simulink model "raspi_MODEL"  (R2022b)
settings: Solver=FixedStepAuto  StartTime=0.0  StopTime=1000  RelTol=1e-3  EnableMultiTasking=on
libraries: raspberrypiBasiclib x6, embedlinuxNetworklib x3, raspberrypiNetworklib x2, raspberrypiAVlib x1
settings Model: SimulationMode=external  Creator=Asus  LastModifiedBy=VIKAS CHEIIURU
settings SolverCC: PositivePriorityOrder=on
settings OptimizationCC: EnhancedBackFolding=on  PassReuseOutputArgsAs=Individual arguments  ZeroExternalMemoryAtStartup=off  ZeroInternalMemoryAtStartup=off  MaxStackSize=64  OptimizeBlockOrder=speed  DifferentSizesBufferReuse=on  OptimizationCustomize=off  EfficientTunableParamExpr=on
settings DebuggingCC: ParameterTunabilityLossMsg=error
settings HardwareCC: ProdBitPerPointer=32  ProdBitPerSizeT=32  ProdBitPerPtrDiffT=32  ProdLargestAtomicInteger=Long  ProdLargestAtomicFloat=Double  ProdWordSize=32  ProdLongLongMode=on  ProdHWDeviceType=ARM Compatible->ARM Cortex
settings RTWCC: Description=Embedded Coder  SystemTargetFile=ert.tlc  HardwareBoard=Raspberry Pi  TemplateMakefile=ert_default_tmf  Toolchain=GNU GCC Embedded Linux  BuildConfiguration=Faster Runs
settings CodeAppCC: ForceParamTrailComments=on  IgnoreCustomStorageClasses=off  OperatorAnnotations=on  SimulinkDataObjDesc=on  SFDataObjDesc=on  InsertBlockDesc=on
settings ERTTargetCC: SupportVariableSizeSignals=on  ExtMode=on  ExtModeTransport=2  ExtModeStaticAlloc=on  ExtModeMexFile=ext_xcp  ExtModeMexArgs='192.168.235.51' 0 17725  ExtModeIntrfLevel=Level2 - Open

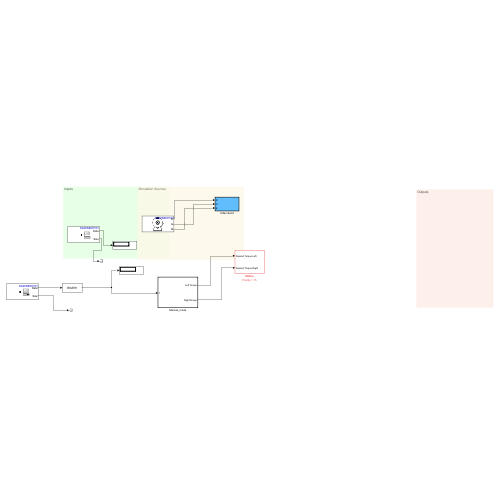
[thumbnail: Simulink's stored preview of the top-level diagram]
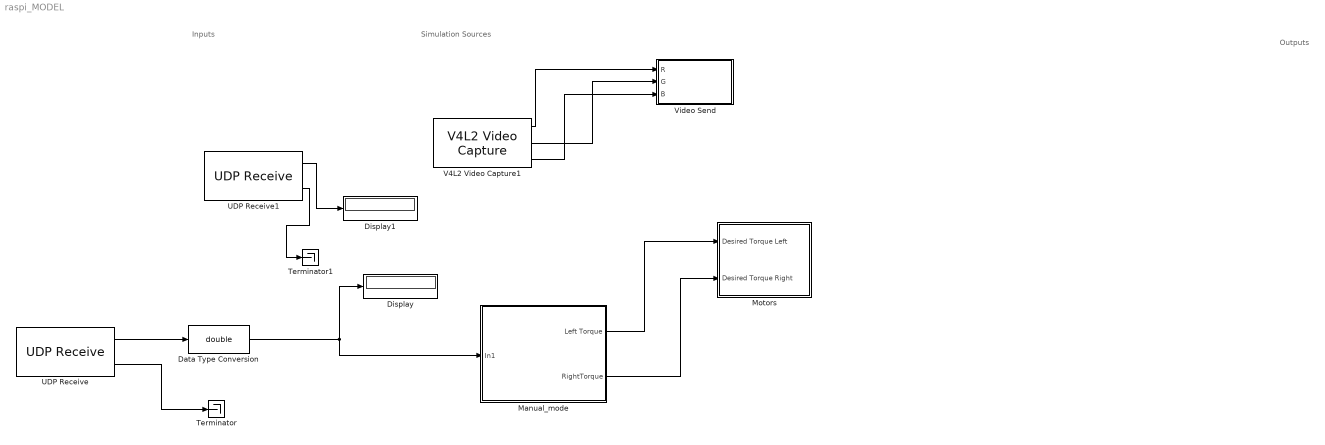
== system raspi_MODEL ==
  note: Inputs
  note: Outputs
  note: Simulation Sources
  Data Type Conversion : DataTypeConversion  OutDataTypeStr=double  RndMeth=Round  SaturateOnIntegerOverflow=off
  Display : Display
  Display1 : Display
  Manual_mode : Subsystem  TreatAsAtomicUnit=on
  Motors : Subsystem  Priority=15
      settings: AttributesFormatString=Priority = %<Priority>
  Terminator : Terminator
  Terminator1 : Terminator
  UDP Receive : raspberrypiNetworklib/UDP Receive  localURL='0.0.0.0'  localPort=26001  remoteURL='0.0.0.0'  remotePort=-1  recvBufferSize=8192  signalDatatype=double  dims=1  isVarSize=off  showBlockingTime=off  blockingTime=0  sampletime=0.01  blockPlatform=Raspberry Pi
  UDP Receive1 : raspberrypiNetworklib/UDP Receive  localURL='0.0.0.0'  localPort=26000  remoteURL='0.0.0.0'  remotePort=-1  recvBufferSize=8192  signalDatatype=boolean  dims=1  isVarSize=off  showBlockingTime=off  blockingTime=0  sampletime=0.01  blockPlatform=Raspberry Pi
  V4L2 Video Capture1 : raspberrypiAVlib/V4L2 Video Capture  DeviceName=/dev/video0  Resolution=160x120  CustomResolution=[ 320, 240 ]  PixelFormat=RGB  SampleTime=0.1  pixelOrder=planar  simOutput=Colorbars  imSizeSelection=320x240  imSize=[640, 480]  roi=[0, 0, 640, 480]  m_devName='/dev/video0'  blockPlatform=LINUX  HorizontalFlip=off  VerticalFlip=off  Brightness=0.5  Saturation=0.5  Contrast=0.5  Sharpness=0.5  CameraPan=0  CameraTilt=0  CameraZoom=0.5  EnableManualFocus=on  ManualFocus=0.5
  Video Send : Subsystem  TreatAsAtomicUnit=on
  wires:
  V4L2 Video Capture1/3 -> Video Send/3(B)
  V4L2 Video Capture1/2 -> Video Send/2(G)
  V4L2 Video Capture1/1 -> Video Send/1(R)
  Manual_mode/2(RightTorque) -> Motors/2(Desired Torque Right)
  Manual_mode/1(Left Torque) -> Motors/1(Desired Torque Left)
  UDP Receive1/1 -> Display1/1
  UDP Receive1/2 -> Terminator1/1
  UDP Receive/1 -> Data Type Conversion/1
  Data Type Conversion/1 -> Manual_mode/1(In1), Display/1
  UDP Receive/2 -> Terminator/1

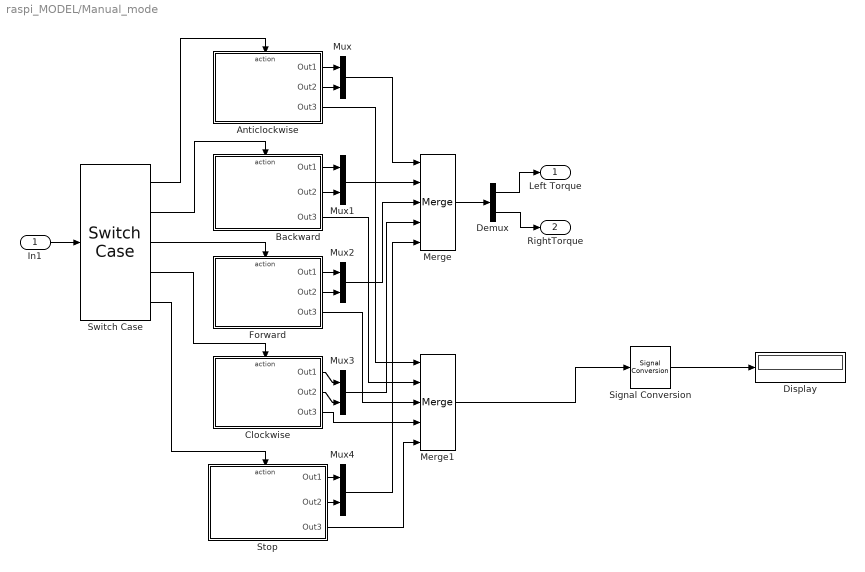
== system raspi_MODEL/Manual_mode ==
  In1 : Inport
  " Anticlockwise" : Subsystem  TreatAsAtomicUnit=on
  Backward : Subsystem  TreatAsAtomicUnit=on
  Clockwise : Subsystem  TreatAsAtomicUnit=on
  Demux : Demux  Outputs=2
  Display : Display
  Forward : Subsystem  TreatAsAtomicUnit=on
  Merge : Merge  Inputs=5
  Merge1 : Merge  Inputs=5  InitialOutput=5
  Mux{,1..4} (5 alike) : Mux  Inputs=2
  Signal Conversion : SignalConversion  OverrideOpt=off
  Stop : Subsystem  TreatAsAtomicUnit=on
  Switch Case : SwitchCase  Priority=1  CaseConditions={2, 3, 4, 5}
      settings: AttributesFormatString=Priority = %<Priority>
  Left Torque : Outport  VectorParamsAs1DForOutWhenUnconnected=off
  RightTorque : Outport  Port=2  VectorParamsAs1DForOutWhenUnconnected=off
  wires:
  Switch Case/1 -> " Anticlockwise"/Action
  Switch Case/2 -> Backward/Action
  Switch Case/3 -> Forward/Action
  Switch Case/4 -> Clockwise/Action
  Switch Case/5 -> Stop/Action
  " Anticlockwise"/2(Out2) -> Mux/2
  " Anticlockwise"/1(Out1) -> Mux/1
  Backward/2(Out2) -> Mux1/2
  Backward/1(Out1) -> Mux1/1
  Forward/2(Out2) -> Mux2/2
  Forward/1(Out1) -> Mux2/1
  Clockwise/1(Out1) -> Mux3/1
  Clockwise/2(Out2) -> Mux3/2
  Stop/1(Out1) -> Mux4/1
  Stop/2(Out2) -> Mux4/2
  Mux2/1 -> Merge/3
  Mux1/1 -> Merge/2
  Mux/1 -> Merge/1
  Mux3/1 -> Merge/4
  Mux4/1 -> Merge/5
  Merge/1 -> Demux/1
  Demux/1 -> Left Torque/1
  Demux/2 -> RightTorque/1
  Stop/3(Out3) -> Merge1/5
  Clockwise/3(Out3) -> Merge1/4
  Forward/3(Out3) -> Merge1/3
  Backward/3(Out3) -> Merge1/2
  " Anticlockwise"/3(Out3) -> Merge1/1
  In1/1 -> Switch Case/1
  Merge1/1 -> Signal Conversion/1
  Signal Conversion/1 -> Display/1

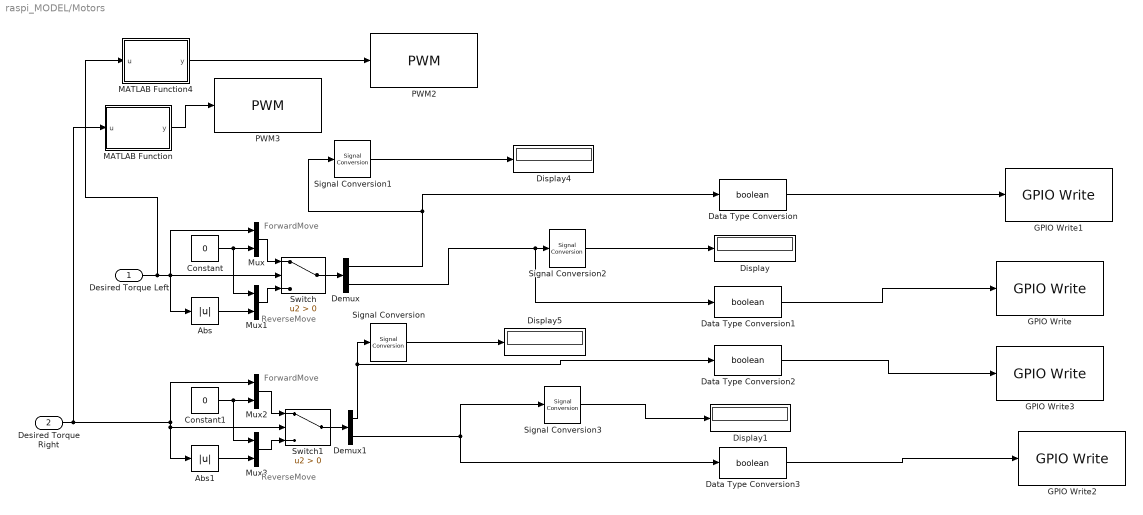
== system raspi_MODEL/Motors ==
  note: ReverseMove
  note: ForwardMove
  note: ReverseMove
  note: ForwardMove
  Desired Torque Left : Inport
  Desired Torque Right : Inport  Port=2
  Abs : Abs  OutDataTypeStr=int16  RndMeth=Round  SaturateOnIntegerOverflow=off
  Abs1 : Abs  OutDataTypeStr=int16  RndMeth=Round  SaturateOnIntegerOverflow=off
  Constant : Constant  Value=0  OutDataTypeStr=int16
  Constant1 : Constant  Value=0  OutDataTypeStr=int16
  Data Type Conversion : DataTypeConversion  OutDataTypeStr=boolean  RndMeth=Nearest  SaturateOnIntegerOverflow=off
  Data Type Conversion1 : DataTypeConversion  OutDataTypeStr=boolean  RndMeth=Round  SaturateOnIntegerOverflow=off
  Data Type Conversion2 : DataTypeConversion  OutDataTypeStr=boolean  RndMeth=Round  SaturateOnIntegerOverflow=off
  Data Type Conversion3 : DataTypeConversion  OutDataTypeStr=boolean  RndMeth=Round  SaturateOnIntegerOverflow=off
  Demux : Demux  Outputs=2
  Demux1 : Demux  Outputs=2
  Display{,1,4..5} (4 alike) : Display
  GPIO Write : raspberrypiBasiclib/GPIO Write  board=Pi 3 Model B  gpio=27  direction=Output  blockPlatform=Raspberry Pi
  GPIO Write1 : raspberrypiBasiclib/GPIO Write  board=Pi 3 Model B  gpio=22  direction=Output  blockPlatform=Raspberry Pi
  GPIO Write2 : raspberrypiBasiclib/GPIO Write  board=Pi 3 Model B  gpio=24  direction=Output  blockPlatform=Raspberry Pi
  GPIO Write3 : raspberrypiBasiclib/GPIO Write  board=Pi 3 Model B  gpio=23  direction=Output  blockPlatform=Raspberry Pi
  MATLAB Function : MATLAB Function  TreatAsAtomicUnit=on
  MATLAB Function4 : MATLAB Function  TreatAsAtomicUnit=on
  Mux{,1..3} (4 alike) : Mux  Inputs=2
  PWM2 : raspberrypiBasiclib/PWM  board=Pi 3 Model B  Pin_=12  Frequency=500  blockPlatform=Raspberry Pi
  PWM3 : raspberrypiBasiclib/PWM  board=Pi 3 Model B  Pin_=13  Frequency=500  blockPlatform=Raspberry Pi
  Signal Conversion{,1..3} (4 alike) : SignalConversion  OverrideOpt=off
  Switch : Switch  Criteria=u2 > Threshold  SaturateOnIntegerOverflow=off  InputSameDT=off
  Switch1 : Switch  Criteria=u2 > Threshold  SaturateOnIntegerOverflow=off  InputSameDT=off
  wires:
  Switch/1 -> Demux/1
  Mux1/1 -> Switch/3
  Constant/1 -> Mux/2, Mux1/1
  Mux/1 -> Switch/1
  Abs/1 -> Mux1/2
  Switch1/1 -> Demux1/1
  Mux3/1 -> Switch1/3
  Constant1/1 -> Mux2/2, Mux3/1
  Abs1/1 -> Mux3/2
  Mux2/1 -> Switch1/1
  Demux/1 -> Data Type Conversion/1, Signal Conversion1/1
  Demux/2 -> Data Type Conversion1/1, Signal Conversion2/1
  Demux1/2 -> Data Type Conversion3/1, Signal Conversion3/1
  Signal Conversion1/1 -> Display4/1
  Desired Torque Right/1 -> Abs1/1, Switch1/2, Mux2/1, MATLAB Function/1(u)
  Desired Torque Left/1 -> MATLAB Function4/1(u), Abs/1, Mux/1, Switch/2
  Signal Conversion/1 -> Display5/1
  Demux1/1 -> Data Type Conversion2/1, Signal Conversion/1
  Signal Conversion2/1 -> Display/1
  Signal Conversion3/1 -> Display1/1
  MATLAB Function/1(y) -> PWM3/1
  MATLAB Function4/1(y) -> PWM2/1
  Data Type Conversion/1 -> GPIO Write1/1
  Data Type Conversion1/1 -> GPIO Write/1
  Data Type Conversion2/1 -> GPIO Write3/1
  Data Type Conversion3/1 -> GPIO Write2/1

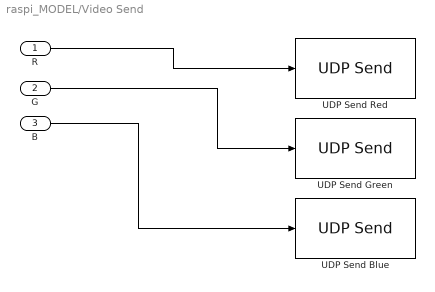
== system raspi_MODEL/Video Send ==
  R : Inport
  G : Inport  Port=2
  B : Inport  Port=3
  UDP Send Blue : embedlinuxNetworklib/UDP Send  remoteURL='255.255.255.255'  remotePort=25002  localURL='255.255.255.255'  localPortSource=Automatically determine  localPort=-1  sampletime=-1  blockPlatform=Raspberry Pi  separateLengthPort=0
  UDP Send Green : embedlinuxNetworklib/UDP Send  remoteURL='255.255.255.255'  remotePort=25001  localURL='255.255.255.255'  localPortSource=Automatically determine  localPort=-1  sampletime=-1  blockPlatform=Raspberry Pi  separateLengthPort=0
  UDP Send Red : embedlinuxNetworklib/UDP Send  remoteURL='255.255.255.255'  remotePort=2500  localURL='255.255.255.255'  localPortSource=Automatically determine  localPort=-1  sampletime=-1  blockPlatform=Raspberry Pi  separateLengthPort=0
  wires:
  R/1 -> UDP Send Red/1
  G/1 -> UDP Send Green/1
  B/1 -> UDP Send Blue/1

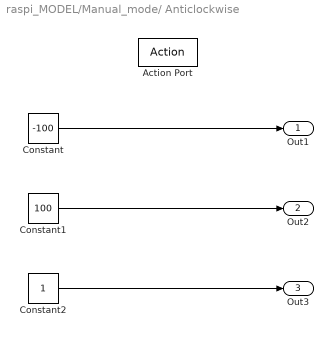
== system raspi_MODEL/Manual_mode/ Anticlockwise ==
  Action Port : ActionPort  ActionPortLabel=case [ 2 ]:
  Constant : Constant  Value=-100  OutDataTypeStr=int16
  Constant1 : Constant  Value=100  OutDataTypeStr=int16
  Constant2 : Constant  OutDataTypeStr=uint8
  Out1 : Outport  InitialOutput=80  VectorParamsAs1DForOutWhenUnconnected=off
  Out2 : Outport  Port=2  InitialOutput=120  VectorParamsAs1DForOutWhenUnconnected=off
  Out3 : Outport  Port=3  InitialOutput=120  VectorParamsAs1DForOutWhenUnconnected=off
  wires:
  Constant/1 -> Out1/1
  Constant1/1 -> Out2/1
  Constant2/1 -> Out3/1

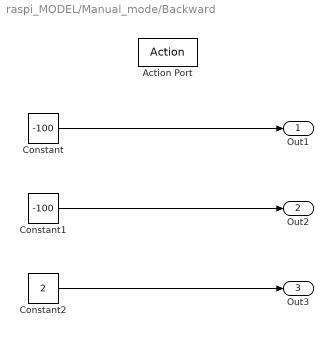
== system raspi_MODEL/Manual_mode/Backward ==
  Action Port : ActionPort  ActionPortLabel=case [ 3 ]:
  Constant : Constant  Value=-100  OutDataTypeStr=int16
  Constant1 : Constant  Value=-100  OutDataTypeStr=int16
  Constant2 : Constant  Value=2  OutDataTypeStr=uint8
  Out1 : Outport  InitialOutput=-100  VectorParamsAs1DForOutWhenUnconnected=off
  Out2 : Outport  Port=2  InitialOutput=-100  VectorParamsAs1DForOutWhenUnconnected=off
  Out3 : Outport  Port=3  InitialOutput=120  VectorParamsAs1DForOutWhenUnconnected=off
  wires:
  Constant/1 -> Out1/1
  Constant1/1 -> Out2/1
  Constant2/1 -> Out3/1

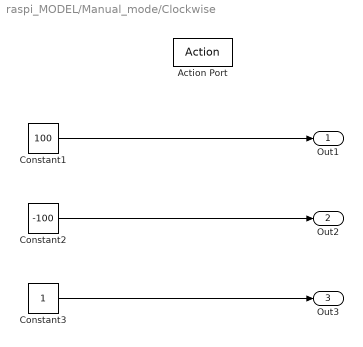
== system raspi_MODEL/Manual_mode/Clockwise ==
  Action Port : ActionPort  ActionPortLabel=case [ 5 ]:
  Constant1 : Constant  Value=100  OutDataTypeStr=int16
  Constant2 : Constant  Value=-100  OutDataTypeStr=int16
  Constant3 : Constant  OutDataTypeStr=uint8
  Out1 : Outport  InitialOutput=0  VectorParamsAs1DForOutWhenUnconnected=off
  Out2 : Outport  Port=2  InitialOutput=0  VectorParamsAs1DForOutWhenUnconnected=off
  Out3 : Outport  Port=3  InitialOutput=120  VectorParamsAs1DForOutWhenUnconnected=off
  wires:
  Constant1/1 -> Out1/1
  Constant2/1 -> Out2/1
  Constant3/1 -> Out3/1

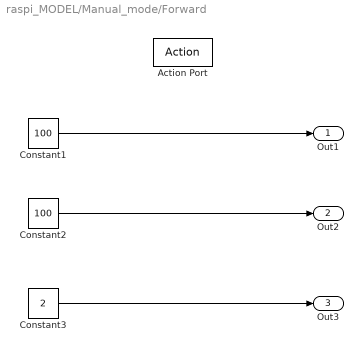
== system raspi_MODEL/Manual_mode/Forward ==
  Action Port : ActionPort  ActionPortLabel=case [ 4 ]:
  Constant1 : Constant  Value=100  OutDataTypeStr=int16
  Constant2 : Constant  Value=100  OutDataTypeStr=int16
  Constant3 : Constant  Value=2  OutDataTypeStr=uint8
  Out1 : Outport  InitialOutput=0  VectorParamsAs1DForOutWhenUnconnected=off
  Out2 : Outport  Port=2  InitialOutput=0  VectorParamsAs1DForOutWhenUnconnected=off
  Out3 : Outport  Port=3  InitialOutput=120  VectorParamsAs1DForOutWhenUnconnected=off
  wires:
  Constant1/1 -> Out1/1
  Constant2/1 -> Out2/1
  Constant3/1 -> Out3/1

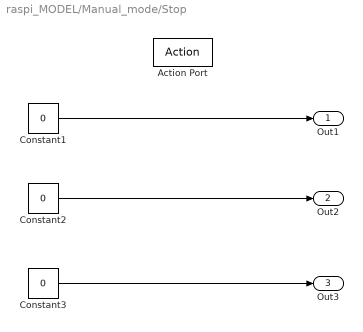
== system raspi_MODEL/Manual_mode/Stop ==
  Action Port : ActionPort  ActionPortLabel=default:
  Constant1 : Constant  Value=0  OutDataTypeStr=int16
  Constant2 : Constant  Value=0  OutDataTypeStr=int16
  Constant3 : Constant  Value=0  OutDataTypeStr=uint8
  Out1 : Outport  InitialOutput=0  VectorParamsAs1DForOutWhenUnconnected=off
  Out2 : Outport  Port=2  InitialOutput=0  VectorParamsAs1DForOutWhenUnconnected=off
  Out3 : Outport  Port=3  InitialOutput=0  VectorParamsAs1DForOutWhenUnconnected=off
  wires:
  Constant1/1 -> Out1/1
  Constant2/1 -> Out2/1
  Constant3/1 -> Out3/1

== matlab function raspi_MODEL/Motors/MATLAB Function4 ==
  data: u input; y output
function y = fcn(u)
y=abs(u);
y =y/100;
end

== matlab function raspi_MODEL/Motors/MATLAB Function ==
  data: u input; y output
function y = fcn(u)
y=abs(u);
y =y/100;
end
